simulink model "campus_windows"  (Simulink 7.9)
settings: Solver=FixedStepDiscrete  StartTime=0.0  StopTime=1*24*60*60  FixedStep=60  RelTol=1e-3
libraries: mlepLibrary x2
settings Model: Creator=willyg  LastModifiedBy=mlab

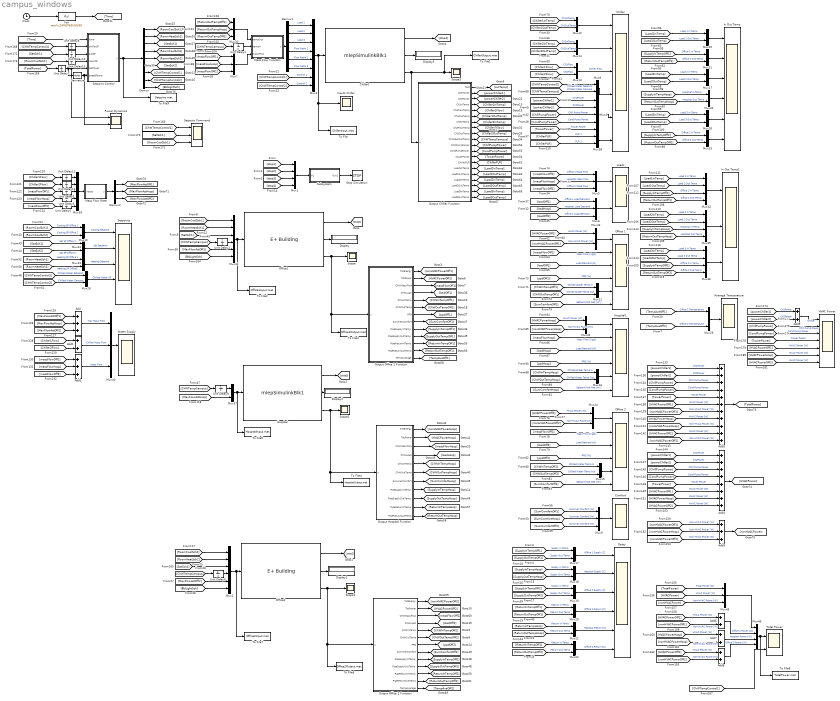
== system campus_windows ==
  Add : Sum  Inputs=+++
  Add{1,6..9} (5 alike) : Sum
  Add2 : Sum  Inputs=+++
  Add3 : Sum  Inputs=+++++++++++
  Add4 : Sum  Inputs=++++++++
  Add5 : Sum  Inputs=+++
  Average Temperature : Scope
      settings: ShowLegends=on  TimeRange=90000  YMin=-0.1  YMax=0.5  SaveName=ScopeData15
  Chiller : Scope  NumInputPorts=6
      settings: ShowLegends=on  TimeRange=90000  YMin=0~0~0~6~0~0  YMax=17.5~17.5~150~17~500000~1  SaveName=ScopeData5
  Chiller1 : M-S-Function  Priority=2  AncestorBlock=mlepLibrary/E+ Building  FunctionName=mlepSimulinkBlk1  Parameters=progname, modelfile, weatherfile, workdir, timeout, port, host, bcvtbdir, deltaT, noutputd  mask(EnergyPlus Cosimulation){progname='C:\\EnergyPlusV8-1-0\\RunEPlus', modelfile='C:\\Users\\mlab\\Documents\\GitRepository\\mlep_v2.0\\CampusSimulation\\Models\\Chiller1\\LargeChiller2', weatherfile='USA_IL_Chicago-OHare.Intl.AP.725300_TMY3', workdir='C:\\Users\\mlab\\Documents\\GitRepository\\mlep_v2.0\\CampusSimulation\\Models\\Chiller1\\', timeout=40000, port=0, host='', bcvtbdir='', deltaT=60, noutputd=20}
      mask prompts: progname "E+ Executable Path"; modelfile "IDF File (without extension)"; weatherfile "Weather Profile"; workdir "Working Directory"; timeout "Timeout (in milliseconds)"; port "Socket Port (0 = any available)"; host "Socket Host ('' = local host)"; bcvtbdir "BCVTB Directory"; deltaT "Time Step (in seconds)"; noutputd "Number of Real Outputs"
      mask help: This block implements cosimulation with EnergyPlus by allowing Simulink to exchange input and output data with it. Currently, EnergyPlus only supports real data.
      mask Help:
      | Simulate a building model using EnergyPlus
      | 
      | <h2>Description</h2>
      | This block implements <a href="http://apps1.eere.energy.gov/buildings/energyplus/">EnergyPlus</a> cosimulation by allowing Simulink to exchange input and output data with EnergyPlus at each time step.
      | 
      | When a simulation starts, this block starts EnergyPlus in parallel. During simulation, EnergyPlus exchanges data with Simulink using the <a href="http://simulationresearch.lbl.gov/bcvtb">Building Controls Virtual Test Bed</a> (BCVTB) interface via <a href="http://mlab.seas.upenn.edu/mlep/">MLE+</a>.
      | 
      | Detailed information about the interface is available in the MLE+ manual.
      | 
      | <h2>Requirements</h2>
      | Requires <a href="http://apps1.eere.energy.gov/buildings/energyplus/">EnergyPlus</a> and <a href="http://mlab.seas.upenn.edu/mlep/">MLE+</a>.
      | 
      | <h2>Input</h2>
      | Block input <b>real</b> is a real vector of EnergyPlus inputs corresponding to the inputs listed in the BCVTB config file <code>variables.cfg</code> (in order).
      | 
      | <h2>Output</h2>
      | The block outputs are, in order:
      | <dl>
      |   <dt><b>flag</b></dt><dd>Status flag for EnergyPlus: 0 if OK, non-zero for error</dd>
      |   <dt><b>time</b></dt><dd>Current simulation time of EnergyPlus (s)</dd>
      |   <dt><b>real</b></dt><dd>Real vector of EnergyPlus outputs corresponding to the outputs listed in the BCVTB config file <code>variables.cfg</code> (in order).</dd>
      | </dl>
      | 
      | <h2>Parameters</h2>
      | The block mask provides inputs for all required MLE+ configuration parameters:
      | <dl>
      |   <dt><b>E+ Executable Path</b></dt><dd>Specify the location of the EnergyPlus executable</dd>
      |   <dt><b>IDF File</b></dt><dd>Specify the EnergyPlus Input Description File (IDF), without extension</dd>
      |   <dt><b>Weather Profile</b></dt><dd>Specify the name of the EnergyPlus weather profile file to use for the model</dd>
      |   <dt><b>Working Directory</b></dt><dd>Specify the EnergyPlus working directory</dd>
      |   <dt><b>Timeout</b></dt><dd>Time delay (ms) before communication between MLE+ and EnergyPlus times out.</dd>
      |   <dt><b>Socket Port</b></dt><dd>Specify the port to use for communicating with EnergyPlus; enter <code>0</code> to use MLE+ default settings.</dd>
      |   <dt><b>Socket Host</b></dt><dd>Specifiy the IP address of the host where EnergyPlus runs; enter <code>''</code> to use localhost (the local computer).</dd>
      |   <dt><b>BCVTB Directory</b></dt><dd>Specify the directory where the BCVTB files reside; enter <code>''</code> to use MLE+ default settings.</dd>
      |   <dt><b>Time Step</b></dt><dd>Enter the EnergyPlus time step (s). This need not be the same as the Simulink time step.</dd>
      |   <dt><b>Number of Real Outputs</b></dt><dd>Specify the number of real outputs from EnergyPlus. This number should match the number of output variables in <code>variables.cfg</code>.</dd>
      | </dl>
      | 
      | All string inputs in the block mask must be passed either as MATLAB strings (that is, surrounded by single quotes <code>'</code>) or as MATLAB expressions which evaluate to strings (for example, <code>[pwd '/somedir']</code>).
      | 
      | <h2>Comments</h2>
      | <ol>
      |   <li>The BCVTB config file <code>variables.cfg</code> must be in the EnergyPlus working directory specified in the block mask.</li>
      |   <li>For fixed time step simulation in Simulink, the EnergyPlus time step should be an exact multiple of the Simulink time step.</li>
      |   <li>For details regarding the implementation of MLE+ and the meaning of the parameters, see the MLE+ <a href="http://mlab.seas.upenn.edu/mlep/">documentation</a>.</li>
      | </ol>
      | 
      | <h2>References</h2>
      | <ol>
      |   <li>W. Bernal, M. Behl, T. X. Nghiem, and R. Mangharam, "MLE+: A Tool for Integrated Design and Deployment of Energy Efficient Building Controls," 4th ACM Workshop On Embedded Sensing Systems For Energy-Efficiency In Buildings, (BuildSys '12), Toronto, Canada, 2012. Available: <a href="http://repository.upenn.edu/mlab_papers/51/">http://repository.upenn.edu/mlab_papers/51/</a></li>
      | </ol>
      mask Display:
      | image(imread('chiller_plant.jpg'))
      | disp('E+\nCosimulation');
      | 
      | % Inputs
      | port_label('input', 1, 'real');
      | 
      | % Outputs
      | port_label('output', 1, 'flag');
      | port_label('output', 2, 'time');
      | port_label('output', 3, 'real');
  Clock : Clock
      settings: Priority=1
  Comfort : Scope
      settings: ShowLegends=on  TimeRange=90000  YMin=-0.1  YMax=0.5  SaveName=ScopeData10
  Delay : Scope  NumInputPorts=6
      settings: ShowLegends=on  TimeRange=90000  YMin=6.7~6.7~6.5~10~8~10  YMax=7~6.9~7.5~16~14~16  SaveName=ScopeData4
  Demux : Demux  Outputs=9
  Demux1 : Demux  Outputs=6
  Demux2 : Demux  Outputs=3
  Derivative : Derivative
  Display{,1..3} (4 alike) : Display
  Fcn : Fcn  Priority=1  Expr=rem(u,24*60*60)/60/60
  HVAC Power : Scope  NumInputPorts=7
      settings: ShowLegends=on  TimeRange=90000  YMin=0~20~-1.5e+06~-1~5~0~-5  YMax=1e+06~60~0~1~15~0.02~5  SaveName=ScopeData20
  Hospital : M-S-Function  Priority=1  AncestorBlock=mlepLibrary/E+ Building  FunctionName=mlepSimulinkBlk1  Parameters=progname, modelfile, weatherfile, workdir, timeout, port, host, bcvtbdir, deltaT, noutputd  mask(EnergyPlus Cosimulation){progname='C:\\EnergyPlusV8-1-0\\RunEPlus', modelfile='C:\\Users\\mlab\\Documents\\GitRepository\\mlep_v2.0\\CampusSimulation\\Models\\Hospital1\\Hospital', weatherfile='USA_IL_Chicago-OHare.Intl.AP.725300_TMY3', workdir='C:\\Users\\mlab\\Documents\\GitRepository\\mlep_v2.0\\CampusSimulation\\Models\\Hospital1\\', timeout=40000, port=0, host='', bcvtbdir='', deltaT=60, noutputd=11}
      mask prompts: progname "E+ Executable Path"; modelfile "IDF File (without extension)"; weatherfile "Weather Profile"; workdir "Working Directory"; timeout "Timeout (in milliseconds)"; port "Socket Port (0 = any available)"; host "Socket Host ('' = local host)"; bcvtbdir "BCVTB Directory"; deltaT "Time Step (in seconds)"; noutputd "Number of Real Outputs"
      mask help: This block implements cosimulation with EnergyPlus by allowing Simulink to exchange input and output data with it. Currently, EnergyPlus only supports real data.
      mask Help:
      | Simulate a building model using EnergyPlus
      | 
      | <h2>Description</h2>
      | This block implements <a href="http://apps1.eere.energy.gov/buildings/energyplus/">EnergyPlus</a> cosimulation by allowing Simulink to exchange input and output data with EnergyPlus at each time step.
      | 
      | When a simulation starts, this block starts EnergyPlus in parallel. During simulation, EnergyPlus exchanges data with Simulink using the <a href="http://simulationresearch.lbl.gov/bcvtb">Building Controls Virtual Test Bed</a> (BCVTB) interface via <a href="http://mlab.seas.upenn.edu/mlep/">MLE+</a>.
      | 
      | Detailed information about the interface is available in the MLE+ manual.
      | 
      | <h2>Requirements</h2>
      | Requires <a href="http://apps1.eere.energy.gov/buildings/energyplus/">EnergyPlus</a> and <a href="http://mlab.seas.upenn.edu/mlep/">MLE+</a>.
      | 
      | <h2>Input</h2>
      | Block input <b>real</b> is a real vector of EnergyPlus inputs corresponding to the inputs listed in the BCVTB config file <code>variables.cfg</code> (in order).
      | 
      | <h2>Output</h2>
      | The block outputs are, in order:
      | <dl>
      |   <dt><b>flag</b></dt><dd>Status flag for EnergyPlus: 0 if OK, non-zero for error</dd>
      |   <dt><b>time</b></dt><dd>Current simulation time of EnergyPlus (s)</dd>
      |   <dt><b>real</b></dt><dd>Real vector of EnergyPlus outputs corresponding to the outputs listed in the BCVTB config file <code>variables.cfg</code> (in order).</dd>
      | </dl>
      | 
      | <h2>Parameters</h2>
      | The block mask provides inputs for all required MLE+ configuration parameters:
      | <dl>
      |   <dt><b>E+ Executable Path</b></dt><dd>Specify the location of the EnergyPlus executable</dd>
      |   <dt><b>IDF File</b></dt><dd>Specify the EnergyPlus Input Description File (IDF), without extension</dd>
      |   <dt><b>Weather Profile</b></dt><dd>Specify the name of the EnergyPlus weather profile file to use for the model</dd>
      |   <dt><b>Working Directory</b></dt><dd>Specify the EnergyPlus working directory</dd>
      |   <dt><b>Timeout</b></dt><dd>Time delay (ms) before communication between MLE+ and EnergyPlus times out.</dd>
      |   <dt><b>Socket Port</b></dt><dd>Specify the port to use for communicating with EnergyPlus; enter <code>0</code> to use MLE+ default settings.</dd>
      |   <dt><b>Socket Host</b></dt><dd>Specifiy the IP address of the host where EnergyPlus runs; enter <code>''</code> to use localhost (the local computer).</dd>
      |   <dt><b>BCVTB Directory</b></dt><dd>Specify the directory where the BCVTB files reside; enter <code>''</code> to use MLE+ default settings.</dd>
      |   <dt><b>Time Step</b></dt><dd>Enter the EnergyPlus time step (s). This need not be the same as the Simulink time step.</dd>
      |   <dt><b>Number of Real Outputs</b></dt><dd>Specify the number of real outputs from EnergyPlus. This number should match the number of output variables in <code>variables.cfg</code>.</dd>
      | </dl>
      | 
      | All string inputs in the block mask must be passed either as MATLAB strings (that is, surrounded by single quotes <code>'</code>) or as MATLAB expressions which evaluate to strings (for example, <code>[pwd '/somedir']</code>).
      | 
      | <h2>Comments</h2>
      | <ol>
      |   <li>The BCVTB config file <code>variables.cfg</code> must be in the EnergyPlus working directory specified in the block mask.</li>
      |   <li>For fixed time step simulation in Simulink, the EnergyPlus time step should be an exact multiple of the Simulink time step.</li>
      |   <li>For details regarding the implementation of MLE+ and the meaning of the parameters, see the MLE+ <a href="http://mlab.seas.upenn.edu/mlep/">documentation</a>.</li>
      | </ol>
      | 
      | <h2>References</h2>
      | <ol>
      |   <li>W. Bernal, M. Behl, T. X. Nghiem, and R. Mangharam, "MLE+: A Tool for Integrated Design and Deployment of Energy Efficient Building Controls," 4th ACM Workshop On Embedded Sensing Systems For Energy-Efficiency In Buildings, (BuildSys '12), Toronto, Canada, 2012. Available: <a href="http://repository.upenn.edu/mlab_papers/51/">http://repository.upenn.edu/mlab_papers/51/</a></li>
      | </ol>
      mask Display:
      | image(imread('building.png'))
      | disp('E+\nCosimulation');
      | 
      | % Inputs
      | port_label('input', 1, 'real');
      | 
      | % Outputs
      | port_label('output', 1, 'flag');
      | port_label('output', 2, 'time');
      | port_label('output', 3, 'real');
  Hospital1 : Scope  NumInputPorts=6
      settings: ShowLegends=on  TimeRange=90000  YMin=0~20~-1500000~-1~5~0  YMax=1000000~60~0~1~15~0.02  SaveName=ScopeData13
  In Out Temp : Scope  NumInputPorts=6
      settings: ShowLegends=on  TimeRange=86400  YMin=6.365~6~6.365~6.5~6.365~6.5  YMax=7.035~14~7.035~10~7.035~11.5  SaveName=ScopeData8
  In Out Temp1 : Scope  NumInputPorts=3
      settings: ShowLegends=on  TimeRange=86400  YMin=6.365~6~6.365  YMax=7.035~14~7.035  SaveName=ScopeData14
  Inputs Chiller : Scope
      settings: ShowLegends=on  TimeRange=90000  YMin=0  YMax=80  SaveName=ScopeData9
  Loads : Scope  NumInputPorts=2
      settings: ShowLegends=on  TimeRange=90000  YMin=0~-3000000  YMax=80~0  SaveName=ScopeData7
  Mass Flow Function : MATLAB Function  Priority=2  TreatAsAtomicUnit=on
  Mass Flow Rate : MATLAB Function  Priority=1  TreatAsAtomicUnit=on
  Mux{1,34..36,46} (5 alike) : Mux
  Mux{8,10..28,31..33,37..38,42..44} (28 alike) : Mux  Inputs=2
  Mux2 : Mux  Inputs=6
  Mux{5..7,9,29..30,40,45} (8 alike) : Mux  Inputs=3
  Mux3 : Mux  Inputs=8
  Mux39 : Mux  Inputs=5
  Mux4 : Mux  Inputs=5
  Mux41 : Mux  Inputs=6
  Office 1 : Scope  NumInputPorts=6
      settings: ShowLegends=on  TimeRange=90000  YMin=0~0~0~-2e+06~0~5  YMax=2e+06~200000~100~0~20~15  SaveName=ScopeData11
  Office 2 : Scope  NumInputPorts=6
      settings: ShowLegends=on  TimeRange=90000  YMin=0~0~0~-2e+06~0~5  YMax=2e+06~200000~100~0~20~15  SaveName=ScopeData12
  Office1 : mlepLibrary/E+ Building  Priority=1  progname='C:\EnergyPlusV8-1-0\RunEPlus'  modelfile='C:\Users\mlab\Documents\GitRepository\mlep_v2.0\CampusSimulation\Models\Office1\LargeOffice'  weatherfile='USA_IL_Chicago-OHare.Intl.AP.725300_TMY3'  workdir='C:\Users\mlab\Documents\GitRepository\mlep_v2.0\CampusSimulation\Models\Office1'  timeout=40000  port=0  host=''  bcvtbdir=''  deltaT=60  noutputd=13
  Office2 : mlepLibrary/E+ Building  Priority=1  progname='C:\EnergyPlusV8-1-0\RunEPlus'  modelfile='C:\Users\mlab\Documents\GitRepository\mlep_v2.0\CampusSimulation\Models\Office2\LargeOffice'  weatherfile='USA_IL_Chicago-OHare.Intl.AP.725300_TMY3'  workdir='C:\Users\mlab\Documents\GitRepository\mlep_v2.0\CampusSimulation\Models\Office2\'  timeout=40000  port=0  host=''  bcvtbdir=''  deltaT=60  noutputd=13
  Output Chiller Function : MATLAB Function  TreatAsAtomicUnit=on
  Output Hospital Function : MATLAB Function  TreatAsAtomicUnit=on
  Output Office 1 Function : MATLAB Function  TreatAsAtomicUnit=on
  Output Office 2 Function : MATLAB Function  TreatAsAtomicUnit=on
  Power Dynamics : Scope  NumInputPorts=2
      settings: ShowLegends=on  TimeRange=90000  YMin=0~-5  YMax=80~5  SaveName=ScopeData17
  Scope{,1..3} (4 alike) : Scope
      Scope settings: YMin=0  YMax=1.4e+09
      Scope1 settings: YMin=0  YMax=1.4e+09
      Scope2 settings: YMin=0  YMax=1.4e+09  SaveName=ScopeData2
      Scope3 settings: YMin=0  YMax=1.4e+09  SaveName=ScopeData3
  Setpoint Command : Scope  NumInputPorts=3
      settings: ShowLegends=on  TimeRange=90000  YMin=0~-5~-5  YMax=80~5~5  SaveName=ScopeData19
  Setpoint Control : MATLAB Function  Priority=1  TreatAsAtomicUnit=on
  Setpoints : Scope  NumInputPorts=5
      settings: ShowLegends=on  TimeRange=90000  YMin=24~11~15~6.7~-1  YMax=27~14~25~7~1  SaveName=ScopeData6
  Stop Simulation : Stop
  Subsystem : Subsystem
  To File : ToFile  Filename=ChillerInput.mat  SaveFormat=Timeseries
  To File1 : ToFile  Filename=ChillerOutput.mat  SaveFormat=Timeseries
  To File2 : ToFile  Filename=Office1Input.mat  SaveFormat=Timeseries
  To File3 : ToFile  Filename=Office1Output.mat  SaveFormat=Timeseries
  To File4 : ToFile  Filename=HospitalOutput.mat  SaveFormat=Timeseries
  To File5 : ToFile  Filename=HospitalInput.mat  SaveFormat=Timeseries
  To File6 : ToFile  Filename=Office2Output.mat  SaveFormat=Timeseries
  To File7 : ToFile  Filename=Office2Input.mat  SaveFormat=Timeseries
  To File8 : ToFile  Filename=TotalPower.mat  SaveFormat=Timeseries
  To File9 : ToFile  Filename=Setpoint.mat  SaveFormat=Timeseries
  Total Power : Scope  NumInputPorts=2
      settings: ShowLegends=on  TimeRange=86400  YMin=0~6.5  YMax=4.75e+06~10  SaveName=ScopeData16
  Unit Delay{1..2,6,9} (4 alike) : UnitDelay  X0=6.7  SampleTime=-1
  Unit Delay{3..5,7..8,10..13} (9 alike) : UnitDelay  Priority=1  SampleTime=-1
  Water Supply : Scope  NumInputPorts=2
      settings: ShowLegends=on  TimeRange=90000  YMin=24~11  YMax=27~14  SaveName=ScopeData18
  wires:
  Office1/2 -> Display/1
  Office1/3 -> Scope/1, Output Office 1 Function/1(u), To File3/1
  Office2/1 -> [stop2]
  Office2/2 -> Display1/1
  Hospital/1 -> [stop3]
  Hospital/2 -> Display2/1
  Hospital/3 -> Scope2/1, Output Hospital Function/1(u), To File4/1
  Office1/1 -> [stop1]
  [stop1] -> Mux1/1
  [stop2] -> Mux1/2
  [stop3] -> Mux1/3
  Mux1/1 -> Subsystem/1(In1)
  Subsystem/1(Out1) -> Stop Simulation/1
  Chiller1/2 -> Display3/1
  Chiller1/3 -> Output Chiller Function/1(u), Scope3/1, To File1/1
  Chiller1/1 -> [stop4]
  Mux3/1 -> Chiller1/1, Inputs Chiller/1, To File/1
  Clock/1 -> Fcn/1
  Fcn/1 -> [Time]
  [stop4] -> Mux1/4
  Office2/3 -> Scope1/1, Output Office 2 Function/1(u), To File6/1
  Setpoint Control/1(y) -> Demux/1, To File9/1
  Demux/1 -> [RoomCoolSch1]
  Demux/2 -> [RoomHeatSch1]
  Demux/3 -> [SatSch1]
  Demux/4 -> [RoomCoolSch2]
  Demux/5 -> [RoomHeatSch2]
  Demux/6 -> [SatSch2]
  [Time] -> Setpoint Control/1(time)
  Demux/7 -> [ChWTempControl1]
  Demux/8 -> [ChWTempControl2]
  Output Chiller Function/1(Tout) -> [outTemp]
  Output Chiller Function/2(Ch1Power) -> [powerChiller1]
  Output Chiller Function/3(Ch2Power) -> [powerChiller2]
  Output Chiller Function/4(Ch1InTemp) -> [Chiller1InTemp]
  Output Chiller Function/5(Ch1FlowTemp) -> [Chiller1Flow]
  Output Chiller Function/6(Ch1OutTemp) -> [Chiller1OutTemp]
  Output Chiller Function/7(Ch2InTemp) -> [Chiller2InTemp]
  Output Chiller Function/8(Ch2FlowTemp) -> [Chiller2Flow]
  Output Chiller Function/9(Ch2OutTemp) -> [Chiller2OutTemp]
  Output Chiller Function/10(ChWaterOutTemp) -> [ChWTempCampus]
  [ChWTempControl1] -> Mux3/7  "Control 1"
  [ChWTempControl2] -> Mux3/8  "Control 2"
  Output Office 1 Function/1(TotEnergy) -> [nonHVACPowerOff1]
  Output Office 1 Function/2(TotPower) -> [HVACPowerOff1]
  Output Office 1 Function/3(ChWMassFlow) -> [massFlowOff1]
  Output Office 1 Function/4(ChWLoad) -> [loadOff1]
  Output Office 1 Function/5(ChWInTemp) -> [ChWInTempOff1]
  Output Office 1 Function/6(ChWOutTemp) -> [ChWOutTempOff1]
  Output Office 1 Function/7(PPD) -> [ppdOff1]
  [massFlowOff1] -> Mux7/1
  Mass Flow Function/1(y) -> Demux1/1
  [massFlowHosp] -> Mux7/2
  [massFlowOff2] -> Mux7/3
  Output Hospital Function/3(ChWMassFlow) -> [massFlowHosp]
  Output Hospital Function/4(ChWLoad) -> [loadHosp]
  Output Hospital Function/5(ChWInTemp) -> [ChWInTempHosp]
  Output Hospital Function/6(ChWOutTemp) -> [ChWOutTempHosp]
  Output Hospital Function/7(SummerComfort) -> [SumComfortHosp]
  Output Office 1 Function/8(SummerComfort) -> [SumComfortOff1]
  [SumComfortOff1] -> Mux9/1  "Summer Comfort [Hr]"
  [SumComfortOff2] -> Mux9/3  "Summer Comfort [Hr]"
  Mux9/1 -> Comfort/1
  [SumComfortHosp] -> Mux9/2  "Summer Comfort [Hr]"
  Output Chiller Function/11(ChillPumpPower) -> [ChillPumpPower]
  [Chiller1InTemp] -> Mux12/1  "Ch1InTemp"
  [Chiller1OutTemp] -> Mux12/2  "Ch1OutTemp"
  [Chiller2InTemp] -> Mux14/1  "Ch2InTemp"
  [Chiller2OutTemp] -> Mux14/2  "Ch2OutTemp"
  Mux12/1 -> Chiller/1
  [Chiller1Flow] -> Mux13/1  "Ch1Flow"
  [Chiller2Flow] -> Mux13/2  "Ch2Flow"
  Mux14/1 -> Chiller/2
  Mux13/1 -> Chiller/3  "Chiller Flow"
  [powerChiller1] -> Mux4/1  "Ch1Power"
  [powerChiller2] -> Mux4/2  "Ch2Power"
  Mux4/1 -> Chiller/5
  [massFlowOff1] -> Mux5/1  "Office 1 Mass Flow"
  [massFlowHosp] -> Mux5/2  "Hospital Mass Flow"
  Mux5/1 -> Loads/1
  [massFlowOff2] -> Mux5/3  "Office 2 Mass Flow"
  [loadOff1] -> Mux6/1  "Office 1 Load Demand"
  [loadHosp] -> Mux6/2  "Hospital Load Demand"
  Mux6/1 -> Loads/2
  [loadOff2] -> Mux6/3  "Office 2 Load Demand"
  [HVACPowerOff1] -> Mux43/1  "HVAC Power [W]"
  [nonHVACPowerOff1] -> Mux43/2  "Non-HVAC Power [W]"
  [massFlowOff1] -> Office 1/2  "Mass Flow [Kg/s]"
  [loadOff1] -> Office 1/3  "Load Demand [W]"
  [ppdOff1] -> Office 1/4  "PPD [%]"
  [ChWInTempOff1] -> Mux11/1  "Chilled Water Temp In"
  [ChWOutTempOff1] -> Mux11/2  "Chilled Water Temp Out"
  Mux11/1 -> Office 1/5
  [SumComfortOff1] -> Office 1/6  "Setpoint Not Met [Hr]"
  [massFlowOff2] -> Office 2/2  "Mass Flow [Kg/s]"
  [loadOff2] -> Office 2/3  "Load Demand [W]"
  [ppdOff2] -> Office 2/4  "PPD [%]"
  [ChWInTempOff2] -> Mux15/1  "Chilled Water Temp In"
  [ChWOutTempOff2] -> Mux15/2  "Chilled Water Temp Out"
  Mux15/1 -> Office 2/5
  [SumComfortOff2] -> Office 2/6  "Setpoint Not Met [Hr]"
  [massFlowHosp] -> Hospital1/2  "Mass Flow [Kg/s]"
  [loadHosp] -> Hospital1/3  "Load Demand [W]"
  [ppdHosp] -> Hospital1/4  "PPD [%]"
  [ChWInTempHosp] -> Mux16/1  "Chilled Water Temp In"
  [ChWOutTempHosp] -> Mux16/2  "Chilled Water Temp Out"
  Mux16/1 -> Hospital1/5
  [SumComfortHosp] -> Hospital1/6  "Setpoint Not Met [Hr]"
  Output Office 1 Function/9(PipeSupplyInTemp) -> [SupplyInTempOff1]
  Output Office 1 Function/10(PipeSupplyOutTemp) -> [SupplyOutTempOff1]
  Output Office 1 Function/11(PipeReturnInTemp) -> [ReturnInTempOff1]
  Output Office 1 Function/12(PipeReturnOutTemp) -> [ReturnOutTempOff1]
  [SupplyInTempOff1] -> Mux17/1  "Supply In Temp"
  [SupplyOutTempOff1] -> Mux17/2  "Supply Out Temp"
  Mux17/1 -> Delay/1  "Office 1 Supply [C]"
  [SupplyInTempHosp] -> Mux18/1  "Supply In Temp"
  [SupplyOutTempHosp] -> Mux18/2  "Supply Out Temp"
  Mux18/1 -> Delay/2  "Hospital Supply [C]"
  [SupplyInTempOff2] -> Mux19/1  "Supply In Temp"
  [SupplyOutTempOff2] -> Mux19/2  "Supply Out Temp"
  Mux19/1 -> Delay/3  "Office 2 Supply [C]"
  [ReturnInTempOff1] -> Mux20/1  "Return In Temp"
  [ReturnOutTempOff1] -> Mux20/2  "Return Out Temp"
  Mux20/1 -> Delay/4  "Office 1 Return [C]"
  [ReturnInTempHosp] -> Mux21/1  "Return In Temp"
  [ReturnOutTempHosp] -> Mux21/2  "Return Out Temp"
  [ReturnInTempOff2] -> Mux22/1  "Return In Temp"
  [ReturnOutTempOff2] -> Mux22/2  "Return Out Temp"
  Mux21/1 -> Delay/5  "Hospital Return [C]"
  Mux22/1 -> Delay/6  "Office 2 Return [C]"
  Output Hospital Function/8(PipeSupplyInTemp) -> [SupplyInTempHosp]
  Output Hospital Function/9(PipeSupplyOutTemp) -> [SupplyOutTempHosp]
  Output Hospital Function/10(PipeReturnInTemp) -> [ReturnInTempHosp]
  Output Hospital Function/11(PipeReturnOutTemp) -> [ReturnOutTempHosp]
  Output Office 2 Function/3(ChWMassFlow) -> [massFlowOff2]
  Output Office 2 Function/4(ChWLoad) -> [loadOff2]
  Output Office 2 Function/5(ChWInTemp) -> [ChWInTempOff2]
  Output Office 2 Function/6(ChWOutTemp) -> [ChWOutTempOff2]
  Output Office 2 Function/7(PPD) -> [ppdOff2]
  Output Office 2 Function/8(SummerComfort) -> [SumComfortOff2]
  Output Office 2 Function/9(PipeSupplyInTemp) -> [SupplyInTempOff2]
  Output Office 2 Function/10(PipeSupplyOutTemp) -> [SupplyOutTempOff2]
  Output Office 2 Function/11(PipeReturnInTemp) -> [ReturnInTempOff2]
  Output Office 2 Function/12(PipeReturnOutTemp) -> [ReturnOutTempOff2]
  [ChWTempCampus] -> Mux8/2  "Chilled Water Campus"
  [ChWTempControl2] -> Mux8/1  "Chilled Water Setpoint"
  Mux8/1 -> Chiller/4
  [RoomCoolSch1] -> Mux10/1  "Cooling SP Office 1"
  [RoomCoolSch2] -> Mux10/2  "Cooling SP Office 2"
  [SatSch1] -> Mux24/1  "Sat SP Office 1"
  [SatSch2] -> Mux24/2  "Sat SP Office 2"
  Mux10/1 -> Setpoints/1  "Cooling Setpoint"
  [RoomHeatSch1] -> Mux23/1  "Heating SP Office 1"
  [RoomHeatSch2] -> Mux23/2  "Heating SP Office2"
  Mux24/1 -> Setpoints/2  "Sat Setpoint"
  Mux23/1 -> Setpoints/3  "Heating Setpoint"
  [ChWTempControl2] -> Mux26/2  "Chilled Water Campus"
  [ChWTempControl1] -> Mux26/1  "Chilled Water Setpoint"
  Mux26/1 -> Setpoints/4  "Chilled Water SP"
  Output Chiller Function/12(CondPumpPower) -> [CondPumpPower]
  Output Chiller Function/13(TowerPower) -> [TowerPower]
  [ChillPumpPower] -> Mux4/3  "Chill Pump Power"
  [CondPumpPower] -> Mux4/4  "Cond Pump Power"
  [TowerPower] -> Mux4/5  "Tower Power"
  Output Chiller Function/14(ChillerPLR) -> [ChillerPLR]
  Output Chiller Function/15(Load1InTemp) -> [Load1InTemp]
  Output Chiller Function/16(Load1OutTemp) -> [Load1OutTemp]
  Output Chiller Function/17(Load2InTemp) -> [Load2InTemp]
  Output Chiller Function/18(Load2OutTemp) -> [Load2OutTemp]
  Output Chiller Function/19(Load3InTemp) -> [Load3InTemp]
  Output Chiller Function/20(Load3OutTemp) -> [Load3OutTemp]
  [Load1InTemp] -> Mux25/1  "Load 1 In Temp"
  [Load1OutTemp] -> Mux25/2  "Load 1 Out Temp"
  Mux25/1 -> In Out Temp/1
  [SupplyInTempOff1] -> Mux31/1  "Office 1 In Temp"
  [ReturnOutTempOff1] -> Mux31/2  "Office 1 Out Temp"
  [Load2InTemp] -> Mux27/1  "Load 2 In Temp"
  [Load2OutTemp] -> Mux27/2  "Load 2 Out Temp"
  [SupplyInTempHosp] -> Mux32/1  "Hospital In Temp"
  [ReturnOutTempHosp] -> Mux32/2  "Hospital Out Temp"
  [Load3InTemp] -> Mux28/1  "Load 3 In Temp"
  [Load3OutTemp] -> Mux28/2  "Load 3 Out Temp"
  [SupplyInTempOff2] -> Mux33/1  "Office 2 In Temp"
  [ReturnOutTempOff2] -> Mux33/2  "Office 2 Out Temp"
  [ReturnOutTempOff1] -> Mux30/1
  [ReturnOutTempHosp] -> Mux30/2
  [ReturnOutTempOff2] -> Mux30/3
  Mux7/1 -> Mass Flow Function/3(massFlow)
  Demux1/1 -> Mux3/1  "Load 1"
  Demux1/2 -> Mux3/2  "Load 2"
  Demux1/3 -> Mux3/3  "Load 3"
  Demux1/4 -> Mux3/4  "Flow Ratio 1"
  Demux1/5 -> Mux3/5  "Flow Ratio 2"
  Demux1/6 -> Mux3/6  "Flow Ratio 3"
  Mux30/1 -> Mass Flow Function/1(tempOut)
  [ChWTempCampus] -> Unit Delay1/1
  Mux31/1 -> In Out Temp/2
  Mux27/1 -> In Out Temp/3
  Mux32/1 -> In Out Temp/4
  Mux28/1 -> In Out Temp/5
  Mux33/1 -> In Out Temp/6
  [Load1InTemp] -> Mux34/1  "Load 1 In Temp"
  [Load1OutTemp] -> Mux34/2  "Load 1 Out Temp"
  Mux34/1 -> In Out Temp1/1
  [SupplyInTempOff1] -> Mux34/3  "Office 1 In Temp"
  [ReturnOutTempOff1] -> Mux34/4  "Office 1 Out Temp"
  [Load2InTemp] -> Mux35/1  "Load 2 In Temp"
  [Load2OutTemp] -> Mux35/2  "Load 2 Out Temp"
  [SupplyInTempHosp] -> Mux35/3  "Hospital In Temp"
  [ReturnOutTempHosp] -> Mux35/4  "Hospital Out Temp"
  [Load3InTemp] -> Mux36/1  "Load 3 In Temp"
  [Load3OutTemp] -> Mux36/2  "Load 3 Out Temp"
  [SupplyInTempOff2] -> Mux36/3  "Office 2 In Temp"
  [ReturnOutTempOff2] -> Mux36/4  "Office 2 Out Temp"
  Mux35/1 -> In Out Temp1/2
  Mux36/1 -> In Out Temp1/3
  Output Office 1 Function/13(TempAverage) -> [TempAveOff1]
  [TempAveOff1] -> Mux29/1  "Office 1 Temperature"
  Mux29/1 -> Average Temperature/1
  Output Office 2 Function/13(TempAverage) -> [TempAveOff2]
  [TempAveOff2] -> Mux29/3  "Office 2 Temperature"
  Mux37/1 -> Hospital/1, To File5/1
  [ChillerPLR] -> Mux38/1  "PLR 1"
  [ChillerPLR] -> Mux38/2  "PLR 2"
  Mux38/1 -> Chiller/6
  Demux2/1 -> [MaxFlowActOff1]
  Demux2/2 -> [MaxFlowActHosp]
  Demux2/3 -> [MaxFlowActOff2]
  Mass Flow Rate/1(y) -> Demux2/1
  [Chiller1Flow] -> Unit Delay11/1
  [Chiller2Flow] -> Unit Delay12/1
  Mux39/1 -> Mass Flow Rate/1(Inputs)
  [massFlowOff1] -> Unit Delay3/1
  [massFlowHosp] -> Unit Delay4/1
  [massFlowOff2] -> Unit Delay5/1
  [MaxFlowActOff1] -> Add/1
  [MaxFlowActHosp] -> Add/2
  [MaxFlowActOff2] -> Add/3
  [Chiller1Flow] -> Add1/1
  [Chiller2Flow] -> Add1/2
  [massFlowOff1] -> Add2/1
  [massFlowHosp] -> Add2/2
  [massFlowOff2] -> Add2/3
  Add/1 -> Mux40/1  "Max Mass Flow"
  Add1/1 -> Mux40/2  "Chiller Mass Flow"
  Add2/1 -> Mux40/3  "Mass Flow"
  Mux40/1 -> Water Supply/1
  Mux41/1 -> Office1/1, To File2/1
  [RoomCoolSch1] -> Mux41/1
  [RoomHeatSch1] -> Mux41/2
  [SatSch1] -> Mux41/3
  [ChWTempCampus] -> Unit Delay2/1
  [MaxFlowActOff1] -> Mux41/5
  Unit Delay2/1 -> Mux41/4
  [ChWTempCampus] -> Unit Delay9/1
  [MaxFlowActHosp] -> Mux37/2
  Unit Delay9/1 -> Mux37/1
  Unit Delay12/1 -> Mux39/2
  Unit Delay11/1 -> Mux39/1
  Unit Delay3/1 -> Mux39/3
  Unit Delay4/1 -> Mux39/4
  Unit Delay5/1 -> Mux39/5
  Unit Delay1/1 -> Mass Flow Function/2(tempIn)
  [powerChiller1] -> Add3/1  "Ch1Power"
  [powerChiller2] -> Add3/2  "Ch2Power"
  [ChillPumpPower] -> Add3/3  "Chill Pump Power"
  [CondPumpPower] -> Add3/4  "Cond Pump Power"
  [TowerPower] -> Add3/5  "Tower Power"
  [HVACPowerOff2] -> Mux44/1  "HVAC Power [W]"
  [nonHVACPowerOff2] -> Mux44/2  "Non-HVAC Power [W]"
  [HVACPowerHosp] -> Mux42/1  "HVAC Power [W]"
  [nonHVACPowerHosp] -> Mux42/2  "Non-HVAC Power [W]"
  Mux43/1 -> Office 1/1
  Mux44/1 -> Office 2/1
  [HVACPowerOff1] -> Add3/6  "HVAC Power [W]"
  [nonHVACPowerOff1] -> Add3/7  "Non-HVAC Power [W]"
  [HVACPowerHosp] -> Add3/8  "HVAC Power [W]"
  [nonHVACPowerHosp] -> Add3/9  "Non-HVAC Power [W]"
  [HVACPowerOff2] -> Add3/10  "HVAC Power [W]"
  [nonHVACPowerOff2] -> Add3/11  "Non-HVAC Power [W]"
  [powerChiller1] -> Add4/1  "Ch1Power"
  [powerChiller2] -> Add4/2  "Ch2Power"
  [ChillPumpPower] -> Add4/3  "Chill Pump Power"
  [CondPumpPower] -> Add4/4  "Cond Pump Power"
  [TowerPower] -> Add4/5  "Tower Power"
  [HVACPowerOff1] -> Add4/6  "HVAC Power [W]"
  [HVACPowerHosp] -> Add4/7  "HVAC Power [W]"
  [HVACPowerOff2] -> Add4/8  "HVAC Power [W]"
  Add3/1 -> [TotalPower]
  [nonHVACPowerOff1] -> Add5/1  "Non-HVAC Power [W]"
  [nonHVACPowerHosp] -> Add5/2  "Non-HVAC Power [W]"
  [nonHVACPowerOff2] -> Add5/3  "Non-HVAC Power [W]"
  Add4/1 -> [HVACPower]
  Add5/1 -> [nonHVACPower]
  Mux45/1 -> Mux46/1
  [TotalPower] -> Mux45/1  "Total Power [W]"
  [HVACPower] -> Mux45/2  "HVAC Power [W]"
  [nonHVACPower] -> Mux45/3  "Non-HVAC Power [W]"
  Mux42/1 -> Hospital1/1
  [HVACPowerOff1] -> Add6/1  "HVAC Power [W]"
  [nonHVACPowerOff1] -> Add6/2  "Non-HVAC Power [W]"
  [HVACPowerHosp] -> Add7/1  "HVAC Power [W]"
  [nonHVACPowerHosp] -> Add7/2  "Non-HVAC Power [W]"
  [HVACPowerOff2] -> Add8/1  "HVAC Power [W]"
  [nonHVACPowerOff2] -> Add8/2  "Non-HVAC Power [W]"
  Add8/1 -> Mux46/4  "Office 2 Power [W]"
  Add7/1 -> Mux46/3  "Hospital Power [W]"
  Add6/1 -> Mux46/2  "Office 1 Power [W]"
  Mux46/1 -> Total Power/1, To File8/1
  Demux/9 -> [BldLightSch]
  [BldLightSch] -> Mux41/6
  Mux2/1 -> Office2/1, To File7/1
  [RoomCoolSch2] -> Mux2/1
  [RoomHeatSch2] -> Mux2/2
  [SatSch2] -> Mux2/3
  [ChWTempCampus] -> Unit Delay6/1
  [MaxFlowActOff2] -> Mux2/5
  Unit Delay6/1 -> Mux2/4
  [BldLightSch] -> Mux2/6
  [TotalPower] -> Unit Delay7/1
  Unit Delay7/1 -> Derivative/1, Setpoint Control/5(totPower), Power Dynamics/1
  Derivative/1 -> Setpoint Control/6(speedPower), Power Dynamics/2
  [ChWTempControl1] -> Total Power/2
  [ChWTempControl1] -> Unit Delay8/1
  Unit Delay8/1 -> Setpoint Control/2(chillerSP)
  [ChWTempControl1] -> Setpoint Command/1
  [SatSch1] -> Setpoint Command/2
  [RoomCoolSch1] -> Setpoint Command/3
  [SatSch1] -> Unit Delay10/1
  [RoomCoolSch1] -> Unit Delay13/1
  Unit Delay10/1 -> Setpoint Control/3(satSP)
  Unit Delay13/1 -> Setpoint Control/4(roomSP)
  Output Office 2 Function/1(TotEnergy) -> [nonHVACPowerOff2]
  Output Office 2 Function/2(TotPower) -> [HVACPowerOff2]
  Output Hospital Function/1(TotEnergy) -> [nonHVACPowerHosp]
  Output Hospital Function/2(TotPower) -> [HVACPowerHosp]
  [powerChiller1] -> Add9/1  "Ch1Power"
  [powerChiller2] -> Add9/2  "Ch2Power"
  [ChillPumpPower] -> HVAC Power/2  "Chill Pump Power"
  [CondPumpPower] -> HVAC Power/3  "Cond Pump Power"
  [TowerPower] -> HVAC Power/4  "Tower Power"
  [HVACPowerOff1] -> HVAC Power/5  "HVAC Power [W]"
  [HVACPowerHosp] -> HVAC Power/6  "HVAC Power [W]"
  [HVACPowerOff2] -> HVAC Power/7  "HVAC Power [W]"
  Add9/1 -> HVAC Power/1  "Chiller"

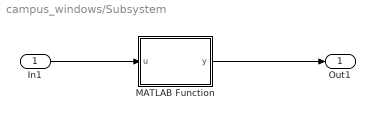
== system campus_windows/Subsystem ==
  In1 : Inport
  MATLAB Function : MATLAB Function  TreatAsAtomicUnit=on
  Out1 : Outport
  wires:
  In1/1 -> MATLAB Function/1(u)
  MATLAB Function/1(y) -> Out1/1

== matlab function Setpoint Control ==
  data: time input double; chillerSP input double; satSP input double; roomSP input double; y output double; totPower input double; speedPower input double
function y = fcn(time, chillerSP, satSP, roomSP, totPower, speedPower)
%#codegen

% Cool
if time < 6
    coolSP = 26.7;
elseif time < 22
    coolSP = 24.0;
else
    coolSP = 26.7;
end

% Heat
if time < 6
    heatSP = 15.6;
elseif time < 22
    heatSP = 21.0;
else
    heatSP = 15.6;
end

% Office 1
RoomCoolSch1 = coolSP;
RoomHeatSch1 = heatSP;
SatSch1 = 12.8;

% Office 2
RoomCoolSch2 = coolSP;
RoomHeatSch2 = heatSP;
SatSch2 = 12.8;

% Chiller
if time < 6
    ChWTempControl1 = 6.7;
    ChWTempControl2 = 6.7;
elseif time < 12
    ChWTempControl1 = 6.7;
    ChWTempControl2 = 6.7;
elseif time < 13
    ChWTempControl1 = 6.7;
    ChWTempControl2 = 6.7;
else
    ChWTempControl1 = 6.7;
    ChWTempControl2 = 6.7;
end

% Light Schedule
if time < 5
    BldLightSch = 0.05;
elseif time < 7
    BldLightSch = 0.1;
elseif time < 8
    BldLightSch = 0.3;
elseif time < 17
    BldLightSch = 0.9;
elseif time < 18
    BldLightSch = 0.7;
elseif time < 20
    BldLightSch = 0.5;
elseif time < 22
    BldLightSch = 0.3;
elseif time < 23
    BldLightSch = 0.1;
else
    BldLightSch = 0.05;
end

%% SELECT CURTAILMENT
% SP 
chillerVar = 1;
satVar = 1;
roomVar = 1;
refPower = 4.1*10^6;
Kp = 7*10^-7;
Kv = -10^-5; % 5*10^-2 -1

% MAX MIN
minChillerV = 6.7;
maxChillerV = 9.44;
minSatV = 12.8;
maxSatV = 15;
minRoomV = 20.6;
maxRoomV = 26.7;

% Time
startTime = 12;
endTime = 16;

%% CHILLER
if chillerVar == 1
    % Reduction
    if time >= startTime && time <= endTime
        
        deltaControl = Kp*(totPower - refPower) + Kv*speedPower; % ChWTempControl1
        if abs(deltaControl) > 0.5
            deltaControl = sign(deltaControl)*0.5;
        end
        
        % Check Chiller
        minV = minChillerV;
        maxV = maxChillerV;
        if chillerSP + deltaControl < minV
            ChWTempControl1 = minV;
        elseif chillerSP + deltaControl > maxV
            ChWTempControl1 = maxV;
        else
            ChWTempControl1 = chillerSP + deltaControl;
        end
    end
    
    ChWTempControl2 = ChWTempControl1;
end
%% SAT
if satVar == 1
    % Reduction
%     Kp = 5*10^-6;

    if time >= startTime && time <= endTime
        
        deltaControl = Kp*(totPower - refPower) + Kv*speedPower; % ChWTempControl1
        if abs(deltaControl) > 0.5
            deltaControl = sign(deltaControl)*0.5;
        end
        
        % Check SAT
        minV = minSatV; % 24.6
        maxV = maxSatV;
        if satSP + deltaControl < minV
            SatSch1 = minV;
        elseif satSP + deltaControl > maxV
            SatSch1 = maxV;
        else
            SatSch1 = satSP + deltaControl;
        end
    end
    
    SatSch2 = SatSch1;
end
%% ROOM
if roomVar == 1
    % Reduction
%     Kp = 10^-6;
%     Kv = 5.10^-2; % 5*10^-2 -1
    if time >= startTime && time <= endTime
        
        deltaControl = Kp*(totPower - refPower) + Kv*speedPower; % ChWTempControl1
        if abs(deltaControl) > 0.5
            deltaControl = sign(deltaControl)*0.5;
        end
        
        % Check ROOM COOL
        minV = minRoomV;
        maxV = maxRoomV;
        if roomSP + deltaControl < minV
            RoomCoolSch1 = minV;
        elseif roomSP  + deltaControl > maxV
            RoomCoolSch1 = maxV;
        else
            RoomCoolSch1 = roomSP + deltaControl;
        end
    end
    
    RoomCoolSch2 = RoomCoolSch1;
end
%%
% Setpoints
y = [RoomCoolSch1 RoomHeatSch1 SatSch1 RoomCoolSch2 RoomHeatSch2 SatSch2 ...
    ChWTempControl1 ChWTempControl2 BldLightSch];

== matlab function Subsystem/MATLAB Function ==
  data: u input double; y output double
function y = fcn(u)
%#codegen
% Number of Inputs
len = length(u);

% Check 
if sum(u==1) == len
    y = 1;
%    y = 0;
else
    y = 0;
end

== matlab function Output Chiller Function ==
  data: u input double; Tout output double; Ch1Power output double; Ch2Power output double; Ch1InTemp output double; Ch1FlowTemp output double; Ch1OutTemp output double; Ch2InTemp output double; Ch2FlowTemp output double; Ch2OutTemp output double; ChWaterOutTemp output double; ChillPumpPower output double; CondPumpPower output double; TowerPower output double; ChillerPLR output double; Load1InTemp output double; Load1OutTemp output double; Load2InTemp output double; Load2OutTemp output double; Load3InTemp output double; Load3OutTemp output double
function [Tout,Ch1Power,Ch2Power,Ch1InTemp,Ch1FlowTemp,Ch1OutTemp,Ch2InTemp,...
    Ch2FlowTemp,Ch2OutTemp,ChWaterOutTemp,ChillPumpPower,CondPumpPower,TowerPower,...
    ChillerPLR,Load1InTemp,Load1OutTemp,Load2InTemp,Load2OutTemp,Load3InTemp,Load3OutTemp] = fcn(u)
%#codegen

% Tout
Tout = u(1);

% Chiller 1 Power
Ch1Power= u(2);
% Chiller 2 Power
Ch2Power = u(3);

% Chiller 1 In Temp
Ch1InTemp = u(4);
% Chiller 1 Flow
Ch1FlowTemp = u(5);
% Chiller 1 Out Temp
Ch1OutTemp = u(6);
% Chiller 2 In Temp
Ch2InTemp = u(7);
% Chiller 2 Flow
Ch2FlowTemp = u(8);
% Chiller 2 Out Temp
Ch2OutTemp = u(9);

% Chillers Out Temp
ChWaterOutTemp = u(10);
% Chiller Pump Temp
ChillPumpPower = u(11);
% Chiller Pump Temp
CondPumpPower = u(12);
% Chiller Pump Temp
TowerPower = u(13);

% Chiller PLR
ChillerPLR = u(14);

% Load 1 In Temp
Load1InTemp = u(15);
% Load 1 Out Temp
Load1OutTemp = u(16);
% Load 2 In Temp
Load2InTemp = u(17);
% Load 2 Out Temp
Load2OutTemp = u(18);
% Load 3 In Temp
Load3InTemp = u(19);
% Load 3 Out Temp
Load3OutTemp = u(20);

% Outputs

== matlab function Output Office 1 Function ==
  data: u input double; TotEnergy output double; TotPower output double; ChWMassFlow output double; ChWLoad output double; ChWInTemp output double; ChWOutTemp output double; PPD output double; SummerComfort output double; PipeSupplyInTemp output double; PipeSupplyOutTemp output double; PipeReturnInTemp output double; PipeReturnOutTemp output double; TempAverage output double
function [TotEnergy,TotPower,ChWMassFlow,ChWLoad,ChWInTemp,ChWOutTemp,PPD,SummerComfort,PipeSupplyInTemp,PipeSupplyOutTemp,PipeReturnInTemp,PipeReturnOutTemp,TempAverage] = fcn(u)
%#codegen

% Total Energy
TotEnergy = u(1);
% Total Power
TotPower = u(2);

% Mass Flow Rate
ChWMassFlow= u(3);
% Heat Transfer Rate
ChWLoad = u(4);

% Chiller 1 In Temp
ChWInTemp = u(5);
% Chiller 1 Flow
ChWOutTemp = u(6);

% Chiller 1 Flow
PPD = u(7);

% Summer Comfort Time
SummerComfort = u(8);

% Pipe Supply In temp
PipeSupplyInTemp = u(9);
% Pipe Supply Out temp
PipeSupplyOutTemp = u(10);
% Pipe Return In temp
PipeReturnInTemp = u(11);
% Pipe Return Out temp
PipeReturnOutTemp = u(12);

% Pipe Return Out temp
TempAverage = u(13);
% Outputs

== matlab function Output Office 2 Function ==
  data: u input double; TotEnergy output double; TotPower output double; ChWMassFlow output double; ChWLoad output double; ChWInTemp output double; ChWOutTemp output double; PPD output double; SummerComfort output double; PipeSupplyInTemp output double; PipeSupplyOutTemp output double; PipeReturnInTemp output double; PipeReturnOutTemp output double; TempAverage output double
function [TotEnergy,TotPower,ChWMassFlow,ChWLoad,ChWInTemp,ChWOutTemp,PPD,SummerComfort,PipeSupplyInTemp,PipeSupplyOutTemp,PipeReturnInTemp,PipeReturnOutTemp,TempAverage] = fcn(u)
%#codegen

% Total Energy
TotEnergy = u(1);
% Total Power
TotPower = u(2);

% Mass Flow Rate
ChWMassFlow= u(3);
% Heat Transfer Rate
ChWLoad = u(4);

% Chiller 1 In Temp
ChWInTemp = u(5);
% Chiller 1 Flow
ChWOutTemp = u(6);

% Chiller 1 Flow
PPD = u(7);

% Summer Comfort Time
SummerComfort = u(8);

% Pipe Supply In temp
PipeSupplyInTemp = u(9);
% Pipe Supply Out temp
PipeSupplyOutTemp = u(10);
% Pipe Return In temp
PipeReturnInTemp = u(11);
% Pipe Return Out temp
PipeReturnOutTemp = u(12);

% Pipe Return Out temp
TempAverage = u(13);
% Outputs

== matlab function Mass Flow Function ==
  data: tempOut input double; tempIn input double; massFlow input double; y output double
function y = fcn(tempOut,tempIn,massFlow)
%#codegen
maxFlow1 = 0.1;
maxFlow2 = 0.06;
maxFlow3 = 0.1;
cp = 4.1855*1000*1.;

% Office 1
flow1 = massFlow(1)/1000;
if flow1 > maxFlow1 
    flow1 = maxFlow1; 
end
ratioFlow1 = flow1/maxFlow1;
load1 = (tempIn - tempOut(1))*massFlow(1)*cp;

% Hospital
flow2 = massFlow(2)/1000;
if flow2 > maxFlow2 
    flow2 = maxFlow2; 
end
ratioFlow2 = flow2/maxFlow2;
load2 = (tempIn - tempOut(2))*massFlow(2)*cp;

% Office 2
flow3 = massFlow(1)/1000;
if flow3 > maxFlow3 
    flow3 = maxFlow3; 
end
ratioFlow3 = flow3/maxFlow3;
load3 = (tempIn - tempOut(3))*massFlow(3)*cp;

y = [load1 load2 load3 ratioFlow1 ratioFlow2 ratioFlow3];

== matlab function Output Hospital Function ==
  data: u input double; TotEnergy output double; TotPower output double; ChWMassFlow output double; ChWLoad output double; ChWInTemp output double; ChWOutTemp output double; SummerComfort output double; PipeSupplyInTemp output double; PipeSupplyOutTemp output double; PipeReturnInTemp output double; PipeReturnOutTemp output double
function [TotEnergy,TotPower,ChWMassFlow,ChWLoad,ChWInTemp,ChWOutTemp,SummerComfort,PipeSupplyInTemp,PipeSupplyOutTemp,PipeReturnInTemp,PipeReturnOutTemp] = fcn(u)
%#codegen

% Total Energy
TotEnergy = u(1);
% Total Power
TotPower = u(2);

% Mass Flow Rate
ChWMassFlow = u(3);
% Heat Transfer Rate
ChWLoad = u(4);

% Chiller 1 In Temp
ChWInTemp = u(5);
% Chiller 1 Flow
ChWOutTemp = u(6);

% Chiller 1 In Temp
SummerComfort = u(7);

% Pipe Supply In temp
PipeSupplyInTemp = u(8);
% Pipe Supply Out temp
PipeSupplyOutTemp = u(9);
% Pipe Return In temp
PipeReturnInTemp = u(10);
% Pipe Return Out temp
PipeReturnOutTemp = u(11);

% Outputs

== matlab function Mass Flow Rate ==
  data: Inputs input double; y output double
function y = fcn(Inputs)
%#codegen

% Chiller Flow
chillerFlow1 = Inputs(1);
chillerFlow2 = Inputs(2);

% Required Flow
massFlowOff1 = Inputs(3);
massFlowHosp = Inputs(4);
massFlowOff2 = Inputs(5);

% Total 
totFlow = chillerFlow1 + chillerFlow2;

% Max Buildings
MaxFlowOff1 = 0.1*1000;
MaxFlowHosp = 0.06*1000;
MaxFlowOff2 = 0.1*1000;

% Remaining  
if massFlowHosp > totFlow
    maxFlowHosp = totFlow;
    remFlow = 0;
else
    maxFlowHosp = massFlowHosp; % massFlowHosp
    remFlow = totFlow - massFlowHosp;
end

% Offices 
% No flow left
if remFlow == 0
    maxFlowOff1 = 0;
    maxFlowOff2 = 0;
% Flow left
else
    % Not enought for both    
    if massFlowOff1 + massFlowOff2 > remFlow
        maxFlowOff1 = remFlow/2;
        maxFlowOff2 = remFlow/2;
    % Enought for both
    else
        maxFlowOff1 = massFlowOff1; % remFlow/2;
        maxFlowOff2 = massFlowOff2; % remFlow/2; %MaxFlowOff2
    end
end

maxFlowOff1 = MaxFlowOff1;
maxFlowHosp = MaxFlowHosp;
maxFlowOff2 = MaxFlowOff2;

% Output
y = [maxFlowOff1 maxFlowHosp maxFlowOff2];
